simulink library "Kl_RFM2G"  (Simulink 7.8)
settings: Solver=ode5  SolverMode=SingleTasking  StartTime=0.0  StopTime=Inf  FixedStep=0.001  RelTol=1e-3
libraries: Rfm2g_syncRecv x1, Rfm2g_init x1, Rfm2g_syncSend x1
settings Model: Creator=pc  LastModifiedBy=pc

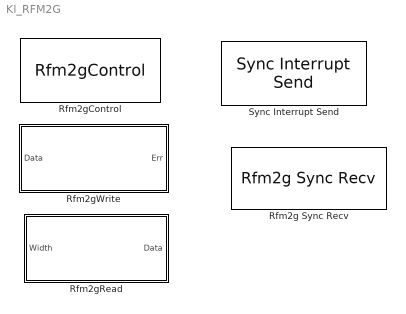
== system Kl_RFM2G ==
  Rfm2g Sync Recv : Rfm2g_syncRecv/Rfm2g Sync Recv  nodeid=0  eventtype=RFM2GEVENT_INTR1  rev0=10  rev1=0
  Rfm2gControl : Rfm2g_init/Rfm2gControl  nodeid=0  rev0=0  rev1=0
  Rfm2gRead : Subsystem  mask(Rfm2g Read){ReadNodeId=0, ReadBufSize=100, ReadOffset=100}
      mask prompts: ReadNodeId "Read From which NodeID"; ReadBufSize "Read Buffer Size (byte)"; ReadOffset "Read Offset"
      mask help:
      | 此模块用于从反射内存卡读取数据,数据读取返回值以字节为单位 .
      |
      | Read From which NodeID
      | 板卡节点号 .
      |
      | read Offset
      | 从偏移地址多少处开始读取数据 ,如偏移 100(十进制) 则填写 100 即可.
      | (实际会从偏移地址处读取 8 个字节数据组成 1 个 double 数据后返回)
      |
      | Width
      | 需要读取的数据的个数,以数组维度表示,如想要读取 2 个数据则可给值 [0 0].
      | Data
      | 返回读取后的 double 数据
      | 读取失败则数据全返回 -1
      mask init:
      | dispblock=sprintf('\nRfm2g Read\n NodeId %d\nOffset 0x%x',ReadNodeId,ReadOffset);
      mask Display: disp(dispblock);
  Rfm2gWrite : Subsystem  mask(Rfm2g Write){WriteNodeId=0, WriteBufSize=100, WriteOffset=100}
      mask prompts: WriteNodeId "Which NodeID to Write"; WriteBufSize "Write Buffer Size (byte)"; WriteOffset "Write Offset"
      mask help:
      | 此模块用于向反射内存卡写数据，数据以字节为单位写入.
      |
      | Which NodeID to Write
      | 板卡节点号．
      |
      | Write Offset
      | 从偏移地址多少处开始写入，如偏移地址　100（十进制）　处开始写入，则填写　100　即可 .
      |
      | Data
      | 需要写入的数据，以 double 格式写入，即一个数据占据　8 个字节存储空间
      | Err
      | 成功返回　0
      | 失败返回 -1
      mask init:
      | dispblock=sprintf('\nRfm2g Write\n NodeID %d\nOffset 0x%x',WriteNodeId,WriteOffset);
      mask Display: disp(dispblock);
  Sync Interrupt Send : Rfm2g_syncSend/Sync Interrupt Send  nodeid=0  towhich=1  eventtype=RFM2GEVENT_INTR1  rev0=0  rev1=0

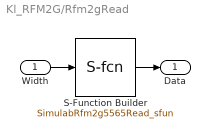
== system Kl_RFM2G/Rfm2gRead ==
  Width : Inport
  S-Function Builder : S-Function  InitFcn=try, set_param(gcb,'FunctionName','SimulabRfm2g5565Read_sfun'), end  FunctionName=SimulabRfm2g5565Read_sfun  Parameters=ReadNodeId,ReadBufSize,ReadOffset  WizardData=DataTag0  EnableBusSupport=off  mask(S-Function Builder){}
      mask help: Simulink:masks:SFunctionBuilder_MD
      mask init:
      | val = [[.9  0.75 0.75 1 1 .9 .9 1]',[1 1 0.75 0.75 .9 .9 1 .9]'];try , sys = get_param(gcb,'SfunBuilderFcnName');if isempty(sys), sys = get_param(gcb,'FunctionName'); end,catch, sys = get_param(gcb,'FunctionName'); end
      settings: CopyFcn=set_param(gcbh,'LinkStatus','none')  PreSaveFcn=try, set_param(gcb,'FunctionName','SimulabRfm2g5565Read_sfun'), end  OpenFcn=sfunctionwizard(gcbh)
      mask Display: plot(val(:,1),val(:,2)),disp(sys), port_label('input',1,'u0'), port_label('output',1,'y0')
  Data : Outport
  wires:
  S-Function Builder/1 -> Data/1
  Width/1 -> S-Function Builder/1

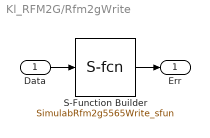
== system Kl_RFM2G/Rfm2gWrite ==
  Data : Inport
  S-Function Builder : S-Function  InitFcn=try, set_param(gcb,'FunctionName','SimulabRfm2g5565Write_sfun'), end  FunctionName=SimulabRfm2g5565Write_sfun  Parameters=WriteNodeId,WriteBufSize,WriteOffset  WizardData=DataTag1  EnableBusSupport=off  mask(S-Function Builder){}
      mask help: Simulink:masks:SFunctionBuilder_MD
      mask init: same as Kl_RFM2G/Rfm2gRead/S-Function Builder
      settings: CopyFcn=set_param(gcbh,'LinkStatus','none')  PreSaveFcn=try, set_param(gcb,'FunctionName','SimulabRfm2g5565Write_sfun'), end  OpenFcn=sfunctionwizard(gcbh)
      mask Display: plot(val(:,1),val(:,2)),disp(sys), port_label('input',1,'u0'), port_label('output',1,'y0')
  Err : Outport
  wires:
  S-Function Builder/1 -> Err/1
  Data/1 -> S-Function Builder/1
